simulink model "lqr_track"  (R2022b)
settings: Solver=VariableStepAuto  StartTime=0.0  StopTime=100.0  RelTol=1e-3
libraries: simulink x1
settings Model: Creator=integzz  LastModifiedBy=integzz

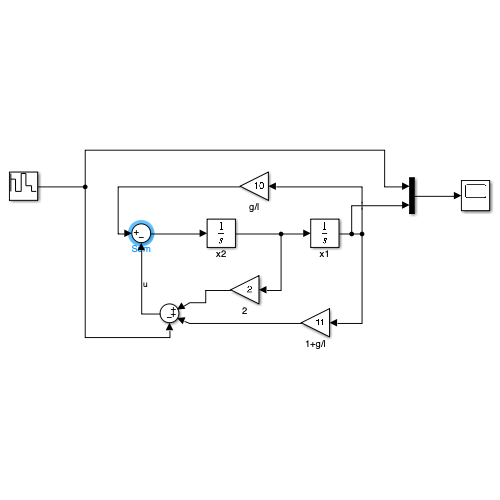
[thumbnail: Simulink's stored preview of the top-level diagram]
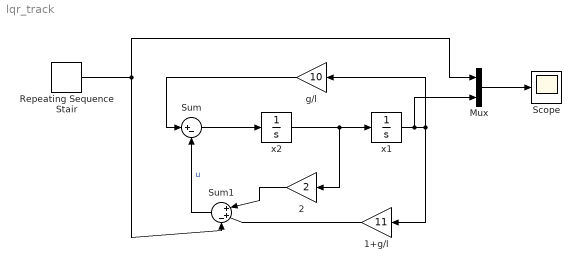
== system lqr_track ==
  1+g/l : Gain  Gain=11
  2 : Gain  Gain=2
  Mux : Mux  Inputs=2
  Repeating Sequence Stair : simulink/Sources/Repeating Sequence Stair  OutValues=[3 1 4 2 1].'  tsamp=20  OutMin=[]  OutMax=[]  OutDataTypeStr=double  OutputDataTypeScalingMode=double  OutDataType=fixdt(0,8)  ConRadixGroup=Best Precision: Vector-wise  OutScaling=2^-12
  Scope : Scope
  Sum : Sum  Inputs=|+-
  Sum1 : Sum  Inputs=|++-
  g/l : Gain  Gain=10
  x1 : Integrator
  x2 : Integrator
  wires:
  x2/1 -> 2/1, x1/1
  x1/1 -> Mux/2, g/l/1, 1+g/l/1
  Sum/1 -> x2/1
  g/l/1 -> Sum/1
  Repeating Sequence Stair/1 -> Sum1/3, Mux/1
  1+g/l/1 -> Sum1/2
  2/1 -> Sum1/1
  Sum1/1 -> Sum/2  "u"
  Mux/1 -> Scope/1
